simulink model "TestDynamicModelRealForce"  (R2022b)
settings: configuration reference "WheelSimConfiguration" (kept outside this file)
settings Model: Creator=At  LastModifiedBy=ateay
settings ConfigSetRef: SourceName=WheelSimConfiguration  SourceLocation=Base Workspace

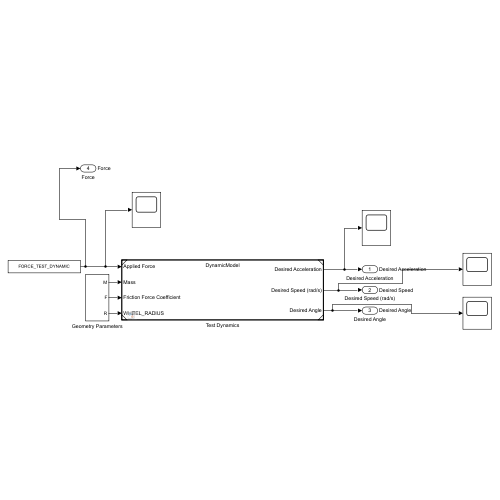
[thumbnail: Simulink's stored preview of the top-level diagram]
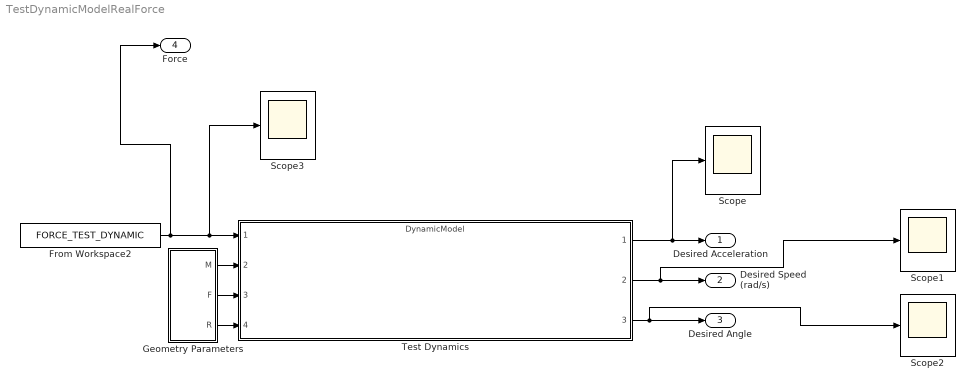
== system TestDynamicModelRealForce ==
  From Workspace2 : FromWorkspace  VariableName=FORCE_TEST_DYNAMIC
  Geometry Parameters : Subsystem  mask{M=90, F=0.0138, rR=0.350}
      mask prompts: M "Mass"; F "Friction"; rR "Radius"
      mask TypeOptions M: Mass/Value
      mask TypeOptions F: Friction/Value
      mask TypeOptions rR: rR/Value
  Scope{,1..3} (4 alike) : Scope
  "Test Dynamics " : ModelReference  ModelNameDialog=DynamicModel.slx  SimulationMode=Normal  ModelReferenceVersion=1.2
  Desired Acceleration : Outport  SignalName=Desired Acceleration
  Desired Speed (rad/s) : Outport  Port=2  SignalName=Desired Speed
  Desired Angle : Outport  Port=3  SignalName=Desired Angle
  Force : Outport  Port=4  SignalName=Force
  wires:
  From Workspace2/1 -> Force/1, Scope3/1, "Test Dynamics "/1
  "Test Dynamics "/3 -> Scope2/1, Desired Angle/1
  "Test Dynamics "/2 -> Scope1/1, Desired Speed (rad/s)/1
  "Test Dynamics "/1 -> Scope/1, Desired Acceleration/1
  Geometry Parameters/1(M) -> "Test Dynamics "/2
  Geometry Parameters/2(F) -> "Test Dynamics "/3
  Geometry Parameters/3(R) -> "Test Dynamics "/4

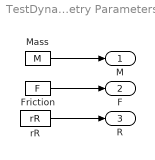
== system TestDynamicModelRealForce/Geometry Parameters ==
  Friction : Constant  Value=F
  Mass : Constant  Value=M
  rR : Constant  Value=rR
  M : Outport
  F : Outport  Port=2
  R : Outport  Port=3
  wires:
  Friction/1 -> F/1
  Mass/1 -> M/1
  rR/1 -> R/1
